simulink model "FC_GPS_FaultModel"  (R2026a)
settings: Solver=FixedStepAuto  StopTime=15  EnableMultiTasking=on
settings Model: Creator=aylin.edgu  LastModifiedBy=aylin.edgu
settings DebuggingCC: InheritedTsInSrcMsg=none

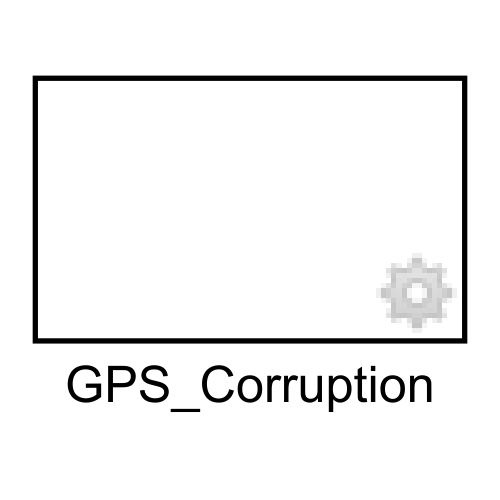
[thumbnail: Simulink's stored preview of the top-level diagram]
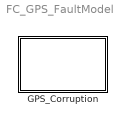
== system FC_GPS_FaultModel ==
  GPS_Corruption : Subsystem  TreatAsAtomicUnit=on  IsInjectorSS=on

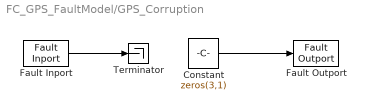
== system FC_GPS_FaultModel/GPS_Corruption ==
  Constant : Constant  Value=zeros(3,1)  SampleTime=-1
  Fault Inport : FaultInport
  Fault Outport : FaultOutport
  Terminator : Terminator
  wires:
  Constant/1 -> Fault Outport/1
  Fault Inport/1 -> Terminator/1
